simulink model "mpc_simulation_2021b"  (R2021b)
settings: Solver=VariableStepAuto  StartTime=0.0  StopTime=5  RelTol=1e-3
undefined symbols (not defined in the file or in its folder): MPCparams
libraries: cstblocks x2
settings Model: Creator=liaml  LastModifiedBy=liamligthart
settings DebuggingCC: UnconnectedInputMsg=none  UnconnectedOutputMsg=none  UnconnectedLineMsg=none
settings ModelReferenceCC: EnableRefExpFcnMdlSchedulingChecks=off
settings RTWCC: DLArmComputeVersion=20.02.1

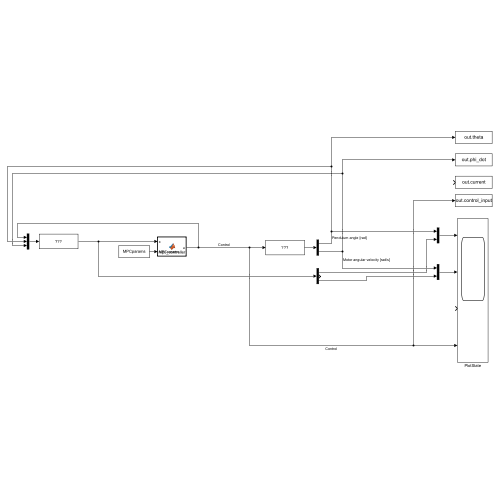
[thumbnail: Simulink's stored preview of the top-level diagram]
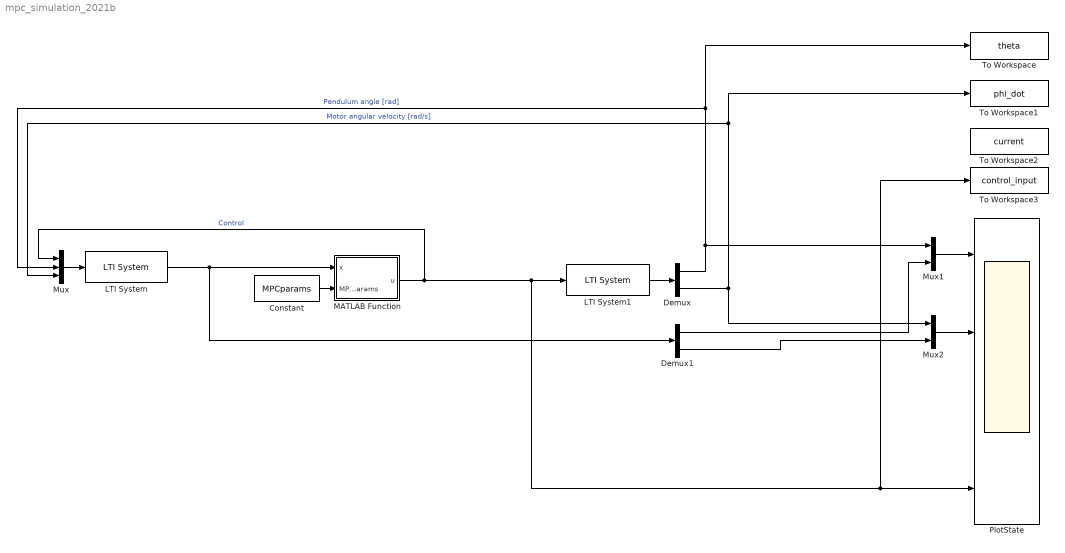
== system mpc_simulation_2021b ==
  Constant : Constant  Value=MPCparams  OutDataTypeStr=Bus: MPCparams_bus
  Demux : Demux  Outputs=2
  Demux1 : Demux  Outputs=3
  LTI System : cstblocks/LTI System  sys=LBGobs  IC=[]
  LTI System1 : cstblocks/LTI System  sys=System  IC=[0.1, 0, 0]
  MATLAB Function : MATLAB Function  TreatAsAtomicUnit=on
  Mux : Mux  Inputs=3
  Mux1 : Mux  Inputs=2
  Mux2 : Mux  Inputs=2
  PlotState : Scope  NumInputPorts=4
  To Workspace : ToWorkspace  VariableName=theta  SaveFormat=Timeseries  SampleTime=-1
  To Workspace1 : ToWorkspace  VariableName=phi_dot  SaveFormat=Timeseries  SampleTime=-1
  To Workspace2 : ToWorkspace  VariableName=current  SaveFormat=Timeseries  SampleTime=-1
  To Workspace3 : ToWorkspace  VariableName=control_input  SaveFormat=Timeseries  SampleTime=-1
  wires:
  MATLAB Function/1(u) -> Mux/1, LTI System1/1, To Workspace3/1, PlotState/4  "Control"
  LTI System/1 -> Demux1/1, MATLAB Function/1(x)
  Constant/1 -> MATLAB Function/2(MPCparams)
  Demux/2 -> To Workspace1/1, Mux/3, Mux2/1  "Motor angular velocity [rad/s]"
  Mux/1 -> LTI System/1
  Demux/1 -> To Workspace/1, Mux/2, Mux1/1  "Pendulum angle [rad]"
  LTI System1/1 -> Demux/1
  Mux1/1 -> PlotState/1
  Mux2/1 -> PlotState/2
  Demux1/1 -> Mux1/2
  Demux1/3 -> Mux2/2

== matlab function mpc_simulation_2021b/MATLAB Function ==
  data: x input; u output; MPCparams input
function u = mpc_controller(x, MPCparams)
    % Inputs:
    % x:            observer state at current time [nx x 1]
    % MPCparams:    struct with all offline MPC calculations
    %
    % Outputs:
    % u:            optimal input at current time [1 x 1]
    
    % Initialize u
    u = zeros(1,1);

    % Compute linear part of cost function (dependent on x0)
    f_i = MPCparams.CostMatrices.f * x;

    % Compute bound vector on u (dependent on x0)
    b_i = [MPCparams.Bounds.bx - MPCparams.Bounds.Ax * MPCparams.PredMatrices.T * x; MPCparams.Bounds.bu];
    
    % Do the optimization
    %coder.extrinsic('quadprog');
    [u_opt, ~, exitflag, ~] = quadprog(MPCparams.CostMatrices.H, f_i, MPCparams.Bounds.A, b_i, [], [], [], [], zeros(size(f_i)), optimoptions('quadprog', Display='off', Algorithm='active-set'));

    if exitflag ~= 1
        disp("WARNING: exitflag = " + exitflag);
    end

    u = u_opt(1);

end
